simulink model "DCS1"  (R2018b)
settings: Solver=VariableStepAuto  StartTime=0.0  StopTime=10.0  RelTol=1e-3
settings Model: Creator=ohara  LastModifiedBy=ohara

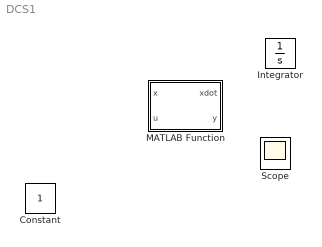
== system DCS1 ==
  Constant : Constant
  Integrator : Integrator
  MATLAB Function : MATLAB Function  TreatAsAtomicUnit=on
  Scope : Scope

== matlab function DCS1/MATLAB Function ==
  data: x input; xdot output; u input; y output
function [xdot, y] = DCS( x, u )
a = 4;
b = 1;
xdot1 = x(2);
xdot2 = -a*x(2)+u;
xdot  = [xdot1; xdot2];
y = x(1);
